simulink library "FMmodelBasic"  (R2022b)
settings: Solver=ode45  StartTime=0.0  StopTime=10.0  RelTol=1e-3  EnableMultiTasking=on
undefined symbols (not defined in the file or in its folder): aeroDB, envDB
libraries: utils x1
(part 1 of 2)
settings Model: Creator=Meyer-Brügel  LastModifiedBy=monas
settings SolverCC: AlgebraicLoopSolver=TrustRegion
settings DataIOCC: LimitDataPoints=on  SaveFormat=Array  ReturnWorkspaceOutputs=off
settings OptimizationCC: LifeSpan=inf
settings DebuggingCC: SolverPrmCheckMsg=warning  UnconnectedInputMsg=warning  UnconnectedOutputMsg=warning  UnconnectedLineMsg=warning  SFUnexpectedBacktrackingDiag=warning  SFNoUnconditionalDefaultTransitionDiag=warning  SFExecutionAtInitializationDiag=none  SFMachineParentedDataDiag=warning  ArithmeticOperatorsInVariantConditions=warning
settings HardwareCC: ProdBitPerPointer=32  ProdBitPerSizeT=32  ProdBitPerPtrDiffT=32  ProdLargestAtomicFloat=None  ProdIntDivRoundTo=Undefined  ProdEndianess=Unspecified  ProdWordSize=32  ProdHWDeviceType=32-bit Generic
settings ModelReferenceCC: EnableRefExpFcnMdlSchedulingChecks=on  PropagateSignalLabelsOutOfModel=off
settings SFSimCC: SimUseLocalCustomCode=off  CustomCodeUndefinedFunction=UseInterfaceOnly
settings RTWCC: RTWUseLocalCustomCode=off  DLArmComputeVersion=19.05
settings CodeAppCC: StateflowObjectComments=on
settings GRTTargetCC: TargetLangStandard=C89/C90 (ANSI)
settings ConfigComp: CovMetricSettings=dw  CovSaveCumulativeToWorkspaceVar=on  CovSaveSingleToWorkspaceVar=on  CovExternalEMLEnable=off  CovSFcnEnable=off

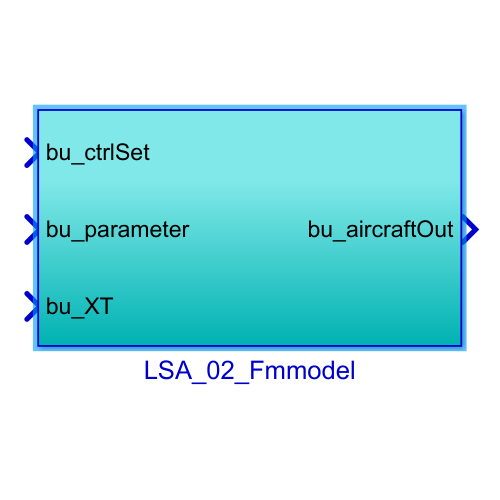
[thumbnail: Simulink's stored preview of the top-level diagram]
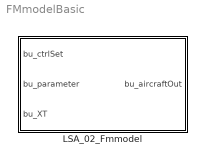
== system FMmodelBasic ==
  LSA_02_Fmmodel : Subsystem

== system FMmodelBasic/LSA_02_Fmmodel ==
  bu_ctrlSet : Inport  OutDataTypeStr=Bus: bu_ctrlSet
  bu_parameter : Inport  Port=2  OutDataTypeStr=Bus: bu_parameter
  bu_XT : Inport  Port=3  OutDataTypeStr=Bus: bu_XT
  Bus Creator : BusCreator  Inputs=3
  aircraft : Subsystem
  integrationProcces : Subsystem
  bu_aircraftOut : Outport  OutDataTypeStr=Bus: bu_aircraftOut
  wires:
  aircraft/1(bu_XaircraftDot) -> integrationProcces/2(bu_XaircraftDot), Bus Creator/2  "bu_XaircraftDot"
  aircraft/2(bu_aircraft) -> Bus Creator/3  "bu_aircraft"
  bu_ctrlSet/1 -> aircraft/2(bu_ctrlSet)
  integrationProcces/1("bu_Xaircraft ") -> aircraft/1("bu_Xaircraft "), Bus Creator/1  "bu_Xaircraft"
  Bus Creator/1 -> bu_aircraftOut/1  "bu_aircraftOut"
  bu_parameter/1 -> aircraft/3(bu_parameter)
  bu_XT/1 -> integrationProcces/1(bu_XT)

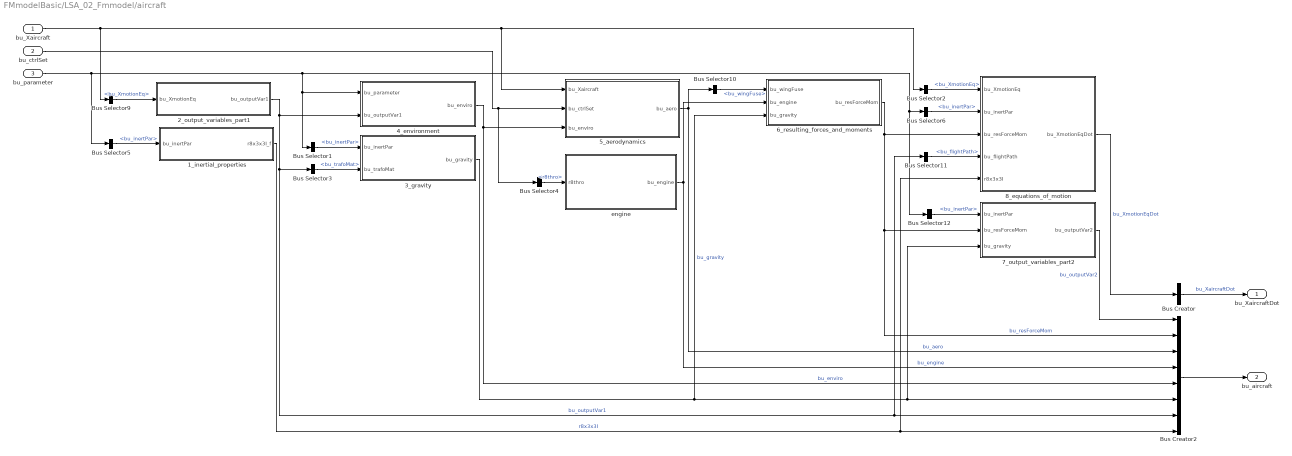
== system FMmodelBasic/LSA_02_Fmmodel/aircraft ==
  "bu_Xaircraft " : Inport
  bu_ctrlSet : Inport  Port=2
  bu_parameter : Inport  Port=3
  1_inertial_properties : Subsystem
  2_output_variables_part1 : Subsystem
  3_gravity : Subsystem
  4_environment : Subsystem
  5_aerodynamics : Subsystem
  6_resulting_forces_and_moments : Subsystem
  7_output_variables_part2 : Subsystem
  8_equations_of_motion : Subsystem
  Bus Creator : BusCreator  Inputs=1
  Bus Creator2 : BusCreator  Inputs=8
  Bus Selector{1,5..6,12} (4 alike) : BusSelector  OutputSignals=bu_inertPar
  Bus Selector10 : BusSelector  OutputSignals=bu_wingFuse
  Bus Selector11 : BusSelector  OutputSignals=bu_flightPath
  Bus Selector2 : BusSelector  OutputSignals=bu_XmotionEq
  Bus Selector3 : BusSelector  OutputSignals=bu_trafoMat
  Bus Selector4 : BusSelector  OutputSignals=r8thro
  Bus Selector9 : BusSelector  OutputSignals=bu_XmotionEq
  engine : Subsystem
  bu_XaircraftDot : Outport
  bu_aircraft : Outport  Port=2
  wires:
  Bus Creator/1 -> bu_XaircraftDot/1  "bu_XaircraftDot"
  Bus Creator2/1 -> bu_aircraft/1
  8_equations_of_motion/1(bu_XmotionEqDot) -> Bus Creator/1  "bu_XmotionEqDot"
  7_output_variables_part2/1(bu_outputVar2) -> Bus Creator2/1  "bu_outputVar2"
  6_resulting_forces_and_moments/1(bu_resForceMom) -> 8_equations_of_motion/3(bu_resForceMom), Bus Creator2/2, 7_output_variables_part2/2(bu_resForceMom)  "bu_resForceMom"
  5_aerodynamics/1(bu_aero) -> Bus Creator2/3, Bus Selector10/1  "bu_aero"
  Bus Selector2/1 -> 8_equations_of_motion/1(bu_XmotionEq)  "<bu_XmotionEq>"
  Bus Selector6/1 -> 8_equations_of_motion/2(bu_inertPar)  "<bu_inertPar>"
  Bus Selector10/1 -> 6_resulting_forces_and_moments/1(bu_wingFuse)  "<bu_wingFuse>"
  bu_ctrlSet/1 -> Bus Selector4/1, 5_aerodynamics/2(bu_ctrlSet)
  Bus Selector1/1 -> 3_gravity/1(bu_inertPar)  "<bu_inertPar>"
  Bus Selector3/1 -> 3_gravity/2(bu_trafoMat)  "<bu_trafoMat>"
  bu_parameter/1 -> Bus Selector12/1, Bus Selector6/1, Bus Selector1/1, 4_environment/1(bu_parameter), Bus Selector5/1
  Bus Selector5/1 -> 1_inertial_properties/1(bu_inertPar)  "<bu_inertPar>"
  "bu_Xaircraft "/1 -> Bus Selector9/1, 5_aerodynamics/1(bu_Xaircraft), Bus Selector2/1
  Bus Selector9/1 -> 2_output_variables_part1/1(bu_XmotionEq)  "<bu_XmotionEq>"
  Bus Selector11/1 -> 8_equations_of_motion/4(bu_flightPath)  "<bu_flightPath>"
  Bus Selector12/1 -> 7_output_variables_part2/1(bu_inertPar)  "<bu_inertPar>"
  2_output_variables_part1/1(bu_outputVar1) -> 4_environment/2(bu_outputVar1), Bus Selector3/1, Bus Selector11/1, Bus Creator2/7  "bu_outputVar1"
  3_gravity/1(bu_gravity) -> 6_resulting_forces_and_moments/3(bu_gravity), 7_output_variables_part2/3(bu_gravity), Bus Creator2/6  "bu_gravity"
  4_environment/1(bu_enviro) -> Bus Creator2/5, 5_aerodynamics/3(bu_enviro)  "bu_enviro"
  1_inertial_properties/1(r8x3x3I_f) -> 8_equations_of_motion/5(r8x3x3I), Bus Creator2/8  "r8x3x3I"
  Bus Selector4/1 -> engine/1(r8thro)  "<r8thro>"
  engine/1(bu_engine) -> Bus Creator2/4, 6_resulting_forces_and_moments/2(bu_engine)  "bu_engine"

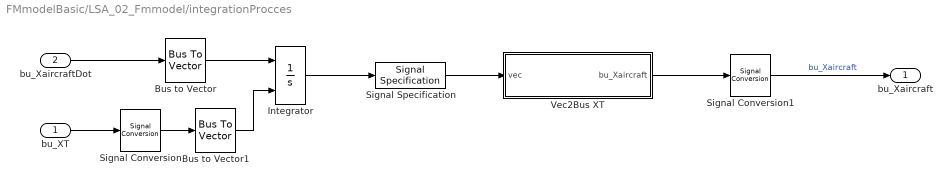
== system FMmodelBasic/LSA_02_Fmmodel/integrationProcces ==
  bu_XT : Inport
  bu_XaircraftDot : Inport  Port=2
  Bus to Vector : BusToVector
  Bus to Vector1 : BusToVector
  Integrator : Integrator  InitialConditionSource=external
  Signal Conversion : SignalConversion  ConversionOutput=Virtual bus  OverrideOpt=off
  Signal Conversion1 : SignalConversion  ConversionOutput=Virtual bus  OverrideOpt=off
  Signal Specification : SignalSpecification  Dimensions=[12,1]
  Vec2Bus XT : MATLAB Function  TreatAsAtomicUnit=on
  "bu_Xaircraft " : Outport
  wires:
  Bus to Vector/1 -> Integrator/1
  Integrator/1 -> Signal Specification/1
  bu_XaircraftDot/1 -> Bus to Vector/1
  bu_XT/1 -> Signal Conversion/1
  Signal Specification/1 -> Vec2Bus XT/1(vec)
  Bus to Vector1/1 -> Integrator/2
  Signal Conversion/1 -> Bus to Vector1/1
  Vec2Bus XT/1(bu_Xaircraft) -> Signal Conversion1/1
  Signal Conversion1/1 -> "bu_Xaircraft "/1  "bu_Xaircraft"

== system FMmodelBasic/LSA_02_Fmmodel/aircraft/1_inertial_properties ==
  bu_inertPar : Inport
  Bus Selector : BusSelector  OutputSignals=r8IOEWxx_f,r8IOEWyy_f,r8IOEWzz_f,r8IOEWxy_f,r8IOEWxz_f,r8IOEWyz_f
  MATLAB Function : MATLAB Function  TreatAsAtomicUnit=on
  r8x3x3I_f : Outport
  wires:
  bu_inertPar/1 -> Bus Selector/1
  Bus Selector/4 -> MATLAB Function/4(r8Ixy_f)  "<r8IOEWxy_f>"
  Bus Selector/6 -> MATLAB Function/6(r8Iyz_f)  "<r8IOEWyz_f>"
  Bus Selector/5 -> MATLAB Function/5(r8Ixz_f)  "<r8IOEWxz_f>"
  Bus Selector/3 -> MATLAB Function/3(r8Izz_f)  "<r8IOEWzz_f>"
  Bus Selector/2 -> MATLAB Function/2(r8Iyy_f)  "<r8IOEWyy_f>"
  Bus Selector/1 -> MATLAB Function/1(r8Ixx_f)  "<r8IOEWxx_f>"
  MATLAB Function/1(r8x3x3I_f) -> r8x3x3I_f/1  "r8x3x3I"

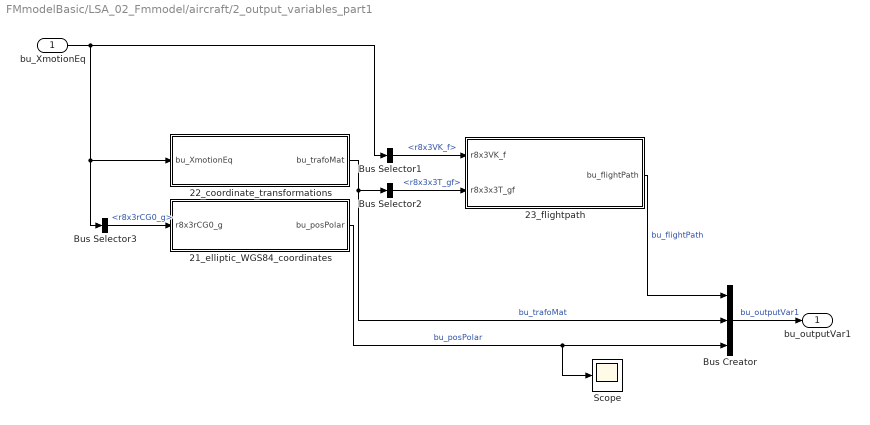
== system FMmodelBasic/LSA_02_Fmmodel/aircraft/2_output_variables_part1 ==
  bu_XmotionEq : Inport
  21_elliptic_WGS84_coordinates : Subsystem
  22_coordinate_transformations : Subsystem
  23_flightpath : Subsystem
  Bus Creator : BusCreator  Inputs=3
  Bus Selector1 : BusSelector  OutputSignals=r8x3VK_f
  Bus Selector2 : BusSelector  OutputSignals=r8x3x3T_gf
  Bus Selector3 : BusSelector  OutputSignals=r8x3rCG0_g
  Scope : Scope
  bu_outputVar1 : Outport
  wires:
  Bus Creator/1 -> bu_outputVar1/1  "bu_outputVar1"
  23_flightpath/1(bu_flightPath) -> Bus Creator/1  "bu_flightPath"
  22_coordinate_transformations/1(bu_trafoMat) -> Bus Creator/2, Bus Selector2/1  "bu_trafoMat"
  bu_XmotionEq/1 -> Bus Selector3/1, 22_coordinate_transformations/1(bu_XmotionEq), Bus Selector1/1
  Bus Selector1/1 -> 23_flightpath/1(r8x3VK_f)  "<r8x3VK_f>"
  Bus Selector2/1 -> 23_flightpath/2(r8x3x3T_gf)  "<r8x3x3T_gf>"
  21_elliptic_WGS84_coordinates/1(bu_posPolar) -> Scope/1, Bus Creator/3  "bu_posPolar"
  Bus Selector3/1 -> 21_elliptic_WGS84_coordinates/1(r8x3rCG0_g)  "<r8x3rCG0_g>"

== system FMmodelBasic/LSA_02_Fmmodel/aircraft/3_gravity ==
  bu_inertPar : Inport
  bu_trafoMat : Inport  Port=2
  31_gravity_g : Subsystem
  32_gravity_f : Subsystem
  Bus Creator1 : BusCreator  Inputs=2
  Bus Selector2 : BusSelector  OutputSignals=r8x3x3T_fg
  Bus Selector3 : BusSelector  OutputSignals=r8mOEW
  bu_gravity : Outport
  wires:
  Bus Creator1/1 -> bu_gravity/1  "bu_gravity"
  Bus Selector3/1 -> 31_gravity_g/1(r8mOEW)  "<r8mOEW>"
  bu_inertPar/1 -> Bus Selector3/1
  Bus Selector2/1 -> 32_gravity_f/1(r8x3x3T_fg)  "<r8x3x3T_fg>"
  bu_trafoMat/1 -> Bus Selector2/1
  32_gravity_f/1(r8x3G_f) -> Bus Creator1/1  "r8x3G_f"
  31_gravity_g/1(r8x3G_g) -> 32_gravity_f/2(r8x3G_g), Bus Creator1/2  "r8x3G_g"

== system FMmodelBasic/LSA_02_Fmmodel/aircraft/4_environment ==
  bu_parameter : Inport
  bu_outputVar1 : Inport  Port=2
  41_atmosphere : Subsystem
  Bus Creator : BusCreator  Inputs=1
  bu_enviro : Outport
  wires:
  Bus Creator/1 -> bu_enviro/1  "bu_enviro"
  41_atmosphere/1(bu_atmos) -> Bus Creator/1  "bu_atmos"
  bu_outputVar1/1 -> 41_atmosphere/2(bu_outputVar1)
  bu_parameter/1 -> 41_atmosphere/1(bu_parameter)

== system FMmodelBasic/LSA_02_Fmmodel/aircraft/5_aerodynamics ==
  bu_Xaircraft : Inport
  bu_ctrlSet : Inport  Port=2
  bu_enviro : Inport  Port=3
  51_effective_flow_at_ARP : Subsystem
  52_wing_and_fuselage : Subsystem
  Bus Creator : BusCreator  Inputs=2
  Bus Selector1 : BusSelector  OutputSignals=bu_XmotionEq
  Bus Selector2 : BusSelector  OutputSignals=bu_XmotionEq
  bu_aero : Outport
  wires:
  52_wing_and_fuselage/1(bu_wingFuse) -> Bus Creator/1  "bu_wingFuse"
  Bus Creator/1 -> bu_aero/1  "bu_aero"
  bu_Xaircraft/1 -> Bus Selector1/1, Bus Selector2/1
  bu_ctrlSet/1 -> 52_wing_and_fuselage/2(bu_ctrlSet)  "bu_ctrlSet"
  Bus Selector1/1 -> 52_wing_and_fuselage/1(bu_XmotionEq)  "<bu_XmotionEq>"
  Bus Selector2/1 -> 51_effective_flow_at_ARP/1(bu_XmotionEq)  "<bu_XmotionEq>"
  51_effective_flow_at_ARP/1(bu_effFlowARP) -> Bus Creator/2, 52_wing_and_fuselage/3(bu_effFlowARP)  "bu_effFlowARP"
  bu_enviro/1 -> 51_effective_flow_at_ARP/2(bu_enviro)

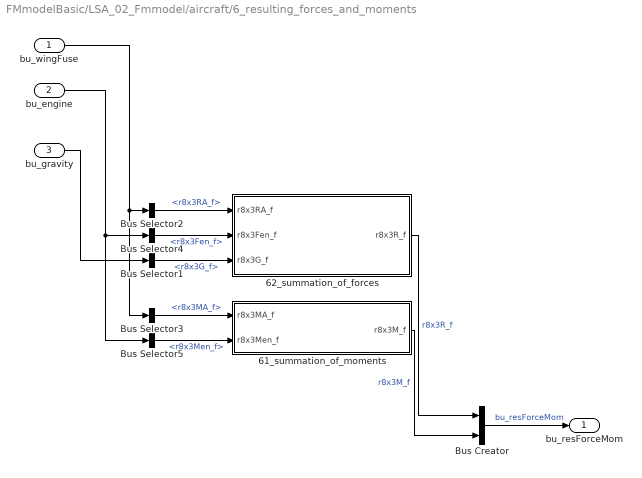
== system FMmodelBasic/LSA_02_Fmmodel/aircraft/6_resulting_forces_and_moments ==
  bu_wingFuse : Inport
  bu_engine : Inport  Port=2
  bu_gravity : Inport  Port=3
  61_summation_of_moments : Subsystem
  62_summation_of_forces : Subsystem
  Bus Creator : BusCreator  Inputs=2
  Bus Selector1 : BusSelector  OutputSignals=r8x3G_f
  Bus Selector2 : BusSelector  OutputSignals=bu_aeroForce.r8x3RA_f
  Bus Selector3 : BusSelector  OutputSignals=bu_aeroMoment.r8x3MA_f
  Bus Selector4 : BusSelector  OutputSignals=r8x3Fen_f
  Bus Selector5 : BusSelector  OutputSignals=r8x3Men_f
  bu_resForceMom : Outport
  wires:
  62_summation_of_forces/1(r8x3R_f) -> Bus Creator/1  "r8x3R_f"
  61_summation_of_moments/1("r8x3M_f ") -> Bus Creator/2  "r8x3M_f"
  Bus Creator/1 -> bu_resForceMom/1  "bu_resForceMom"
  Bus Selector2/1 -> 62_summation_of_forces/1(r8x3RA_f)  "<r8x3RA_f>"
  Bus Selector1/1 -> 62_summation_of_forces/3(r8x3G_f)  "<r8x3G_f>"
  Bus Selector3/1 -> 61_summation_of_moments/1(r8x3MA_f)  "<r8x3MA_f>"
  bu_wingFuse/1 -> Bus Selector3/1, Bus Selector2/1
  bu_gravity/1 -> Bus Selector1/1
  Bus Selector4/1 -> 62_summation_of_forces/2(r8x3Fen_f)  "<r8x3Fen_f>"
  bu_engine/1 -> Bus Selector4/1, Bus Selector5/1
  Bus Selector5/1 -> 61_summation_of_moments/2(r8x3Men_f)  "<r8x3Men_f>"

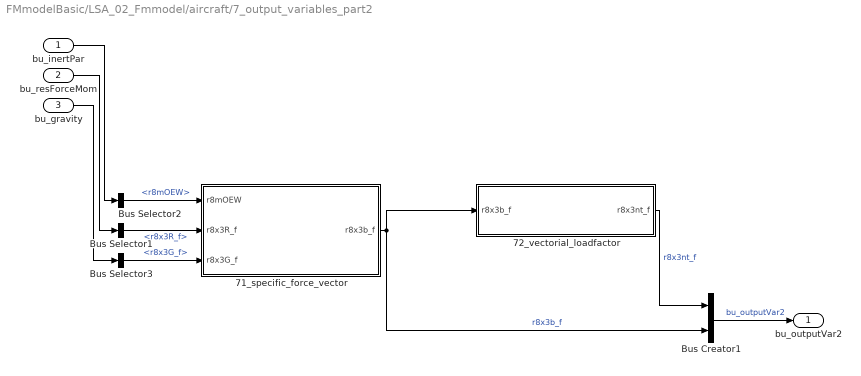
== system FMmodelBasic/LSA_02_Fmmodel/aircraft/7_output_variables_part2 ==
  bu_inertPar : Inport
  bu_resForceMom : Inport  Port=2
  bu_gravity : Inport  Port=3
  71_specific_force_vector : Subsystem
  72_vectorial_loadfactor : Subsystem
  Bus Creator1 : BusCreator  Inputs=2
  Bus Selector1 : BusSelector  OutputSignals=r8x3R_f
  Bus Selector2 : BusSelector  OutputSignals=r8mOEW
  Bus Selector3 : BusSelector  OutputSignals=r8x3G_f
  bu_outputVar2 : Outport
  wires:
  72_vectorial_loadfactor/1(r8x3nt_f) -> Bus Creator1/1  "r8x3nt_f"
  Bus Creator1/1 -> bu_outputVar2/1  "bu_outputVar2"
  Bus Selector2/1 -> 71_specific_force_vector/1(r8mOEW)  "<r8mOEW>"
  Bus Selector1/1 -> 71_specific_force_vector/2(r8x3R_f)  "<r8x3R_f>"
  Bus Selector3/1 -> 71_specific_force_vector/3(r8x3G_f)  "<r8x3G_f>"
  bu_inertPar/1 -> Bus Selector2/1
  bu_resForceMom/1 -> Bus Selector1/1
  bu_gravity/1 -> Bus Selector3/1
  71_specific_force_vector/1(r8x3b_f) -> 72_vectorial_loadfactor/1(r8x3b_f), Bus Creator1/2  "r8x3b_f"

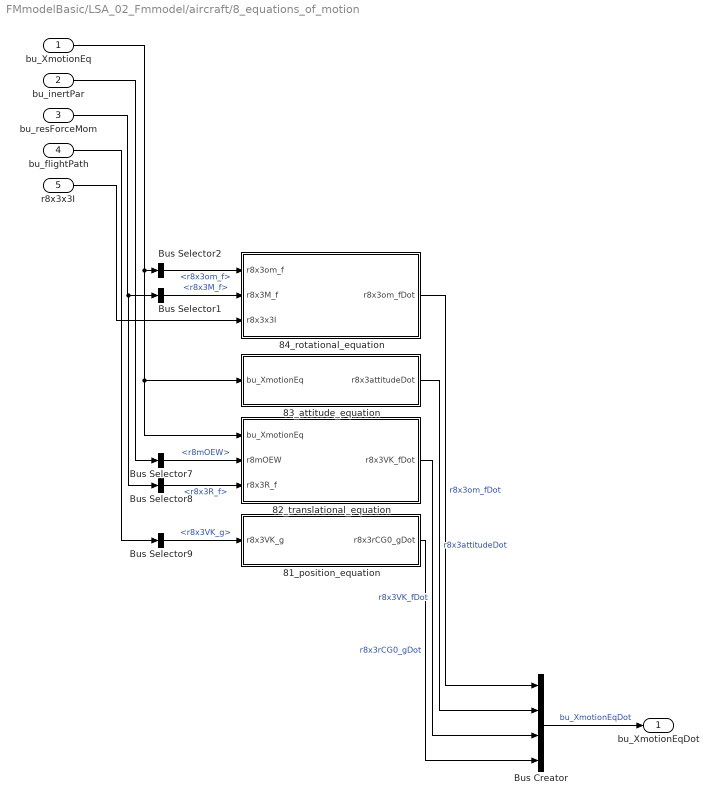
== system FMmodelBasic/LSA_02_Fmmodel/aircraft/8_equations_of_motion ==
  bu_XmotionEq : Inport
  bu_inertPar : Inport  Port=2
  bu_resForceMom : Inport  Port=3
  bu_flightPath : Inport  Port=4
  r8x3x3I : Inport  Port=5
  81_position_equation : Subsystem
  82_translational_equation : Subsystem
  83_attitude_equation : Subsystem
  84_rotational_equation : Subsystem
  Bus Creator : BusCreator  Inputs=4
  Bus Selector1 : BusSelector  OutputSignals=r8x3M_f
  Bus Selector2 : BusSelector  OutputSignals=r8x3om_f
  Bus Selector7 : BusSelector  OutputSignals=r8mOEW
  Bus Selector8 : BusSelector  OutputSignals=r8x3R_f
  Bus Selector9 : BusSelector  OutputSignals=r8x3VK_g
  bu_XmotionEqDot : Outport
  wires:
  Bus Creator/1 -> bu_XmotionEqDot/1  "bu_XmotionEqDot"
  Bus Selector2/1 -> 84_rotational_equation/1(r8x3om_f)  "<r8x3om_f>"
  Bus Selector1/1 -> 84_rotational_equation/2(r8x3M_f)  "<r8x3M_f>"
  bu_XmotionEq/1 -> 82_translational_equation/1(bu_XmotionEq), 83_attitude_equation/1(bu_XmotionEq), Bus Selector2/1
  bu_resForceMom/1 -> Bus Selector8/1, Bus Selector1/1
  r8x3x3I/1 -> 84_rotational_equation/3(r8x3x3I)
  Bus Selector7/1 -> 82_translational_equation/2(r8mOEW)  "<r8mOEW>"
  bu_inertPar/1 -> Bus Selector7/1
  Bus Selector8/1 -> 82_translational_equation/3(r8x3R_f)  "<r8x3R_f>"
  Bus Selector9/1 -> 81_position_equation/1(r8x3VK_g)  "<r8x3VK_g>"
  bu_flightPath/1 -> Bus Selector9/1
  84_rotational_equation/1(r8x3om_fDot) -> Bus Creator/1  "r8x3om_fDot"
  83_attitude_equation/1(r8x3attitudeDot) -> Bus Creator/2  "r8x3attitudeDot"
  82_translational_equation/1(r8x3VK_fDot) -> Bus Creator/3  "r8x3VK_fDot"
  81_position_equation/1(r8x3rCG0_gDot) -> Bus Creator/4  "r8x3rCG0_gDot"

== system FMmodelBasic/LSA_02_Fmmodel/aircraft/engine ==
  r8thro : Inport
  Bus Creator1 : BusCreator  Inputs=2
  Constant : Constant  Value=[1;0;0]  VectorParams1D=off
  Constant1 : Constant  Value=[0;0;0]  VectorParams1D=off
  Product : Product
  bu_engine : Outport
  wires:
  r8thro/1 -> Product/2
  Constant/1 -> Product/1
  Product/1 -> Bus Creator1/1  "r8x3Fen_f"
  Constant1/1 -> Bus Creator1/2  "r8x3Men_f"
  Bus Creator1/1 -> bu_engine/1  "bu_engine"

== system FMmodelBasic/LSA_02_Fmmodel/aircraft/2_output_variables_part1/21_elliptic_WGS84_coordinates ==
  r8x3rCG0_g : Inport
  Bus Creator : BusCreator  Inputs=3
  Demux : Demux  Outputs=3
  Divide : Product  Inputs=/*
  Fcn : Fcn  Expr=cos(u)*envDB.RE
  Gain : Gain  Gain=-1
  Gain1 : Gain  Gain=1/envDB.RE
  bu_posPolar : Outport
  wires:
  r8x3rCG0_g/1 -> Demux/1
  Bus Creator/1 -> bu_posPolar/1  "bu_posPolar"
  Demux/1 -> Gain1/1  "r8x_g"
  Demux/2 -> Divide/2  "r8y_g"
  Demux/3 -> Gain/1  "r8z_g"
  Gain/1 -> Bus Creator/3  "r8Hellip"
  Gain1/1 -> Bus Creator/1, Fcn/1  "r8lat"
  Divide/1 -> Bus Creator/2  "r8lon"
  Fcn/1 -> Divide/1

== system FMmodelBasic/LSA_02_Fmmodel/aircraft/2_output_variables_part1/22_coordinate_transformations ==
  bu_XmotionEq : Inport
  221_geodetic_to_bodyfixed : Subsystem
  222_bodyfixed_to_geodetic : Subsystem
  Bus Creator : BusCreator  Inputs=2
  Bus Selector5 : BusSelector  OutputSignals=r8x3attitude
  bu_trafoMat : Outport
  wires:
  bu_XmotionEq/1 -> Bus Selector5/1
  Bus Creator/1 -> bu_trafoMat/1  "bu_trafoMat"
  Bus Selector5/1 -> 221_geodetic_to_bodyfixed/1(r8x3attitude)  "<r8x3attitude>"
  222_bodyfixed_to_geodetic/1(r8x3x3T_gf) -> Bus Creator/1  "r8x3x3T_gf"
  221_geodetic_to_bodyfixed/1(r8x3x3T_fg) -> 222_bodyfixed_to_geodetic/1(r8x3x3T_fg), Bus Creator/2  "r8x3x3T_fg"

== system FMmodelBasic/LSA_02_Fmmodel/aircraft/2_output_variables_part1/23_flightpath ==
  r8x3VK_f : Inport
  r8x3x3T_gf : Inport  Port=2
  Bus Creator : BusCreator  Inputs=4
  MATLAB Function : MATLAB Function  TreatAsAtomicUnit=on
  Product : Product  Multiplication=Matrix(*)
  bu_flightPath : Outport
  wires:
  Bus Creator/1 -> bu_flightPath/1  "bu_flightPath"
  r8x3x3T_gf/1 -> Product/1
  Product/1 -> Bus Creator/4, MATLAB Function/1(r8x3VK_g)  "r8x3VK_g"
  r8x3VK_f/1 -> Product/2
  MATLAB Function/1(r8VK) -> Bus Creator/1  "r8VK"
  MATLAB Function/2(r8ga) -> Bus Creator/2  "r8ga"
  MATLAB Function/3(r8Ch) -> Bus Creator/3  "r8Ch"

== system FMmodelBasic/LSA_02_Fmmodel/aircraft/3_gravity/31_gravity_g ==
  r8mOEW : Inport
  Product : Product  RndMeth=Zero
  Vector Concatenate : Concatenate  NumInputs=3  Mode=Multidimensional array
  r8XG_g : Constant  Value=0
  r8YG_g : Constant  Value=0
  r8g : Constant  Value=envDB.g
  r8x3G_g : Outport
  wires:
  r8g/1 -> Product/2
  Product/1 -> Vector Concatenate/3
  r8XG_g/1 -> Vector Concatenate/1
  r8YG_g/1 -> Vector Concatenate/2
  r8mOEW/1 -> Product/1
  Vector Concatenate/1 -> r8x3G_g/1  "r8x3G_g"

== system FMmodelBasic/LSA_02_Fmmodel/aircraft/3_gravity/32_gravity_f ==
  r8x3x3T_fg : Inport
  r8x3G_g : Inport  Port=2
  Product1 : Product  Multiplication=Matrix(*)  RndMeth=Zero
  r8x3G_f : Outport
  wires:
  r8x3G_g/1 -> Product1/2
  Product1/1 -> r8x3G_f/1  "r8x3G_f"
  r8x3x3T_fg/1 -> Product1/1

== system FMmodelBasic/LSA_02_Fmmodel/aircraft/4_environment/41_atmosphere ==
  bu_parameter : Inport
  bu_outputVar1 : Inport  Port=2
  411_ISA_conditions : Subsystem
  412_wind : Subsystem
  Bus Creator1 : BusCreator  Inputs=2
  Bus Selector2 : BusSelector  OutputSignals=bu_trafoMat
  Bus Selector3 : BusSelector  OutputSignals=bu_posPolar.r8Hellip
  bu_atmos : Outport
  wires:
  411_ISA_conditions/1(bu_ISA) -> Bus Creator1/2  "bu_ISA"
  412_wind/1(bu_wind) -> Bus Creator1/1  "bu_wind"
  bu_parameter/1 -> 412_wind/1(bu_parameter)
  Bus Selector2/1 -> 412_wind/2(bu_trafoMat)  "<bu_trafoMat>"
  Bus Selector3/1 -> 411_ISA_conditions/1(r8Hellip)  "<r8Hellip>"
  bu_outputVar1/1 -> Bus Selector3/1, Bus Selector2/1
  Bus Creator1/1 -> bu_atmos/1  "bu_atmos"

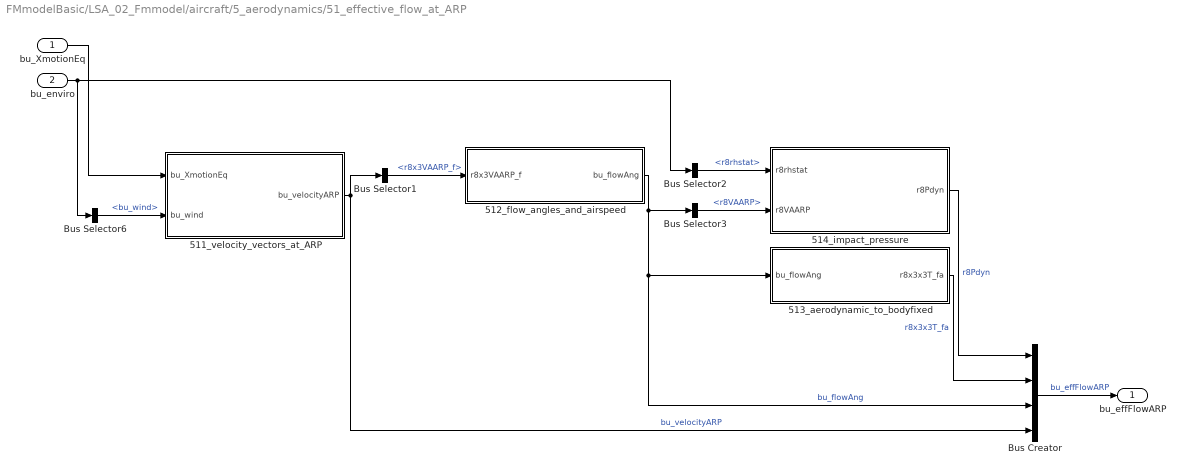
== system FMmodelBasic/LSA_02_Fmmodel/aircraft/5_aerodynamics/51_effective_flow_at_ARP ==
  bu_XmotionEq : Inport
  bu_enviro : Inport  Port=2
  511_velocity_vectors_at_ARP : Subsystem
  512_flow_angles_and_airspeed : Subsystem
  513_aerodynamic_to_bodyfixed : Subsystem
  514_impact_pressure : Subsystem
  Bus Creator : BusCreator  Inputs=4
  Bus Selector1 : BusSelector  OutputSignals=r8x3VAARP_f
  Bus Selector2 : BusSelector  OutputSignals=bu_atmos.bu_ISA.r8rhstat
  Bus Selector3 : BusSelector  OutputSignals=r8VAARP
  Bus Selector6 : BusSelector  OutputSignals=bu_atmos.bu_wind
  bu_effFlowARP : Outport
  wires:
  Bus Creator/1 -> bu_effFlowARP/1  "bu_effFlowARP"
  Bus Selector2/1 -> 514_impact_pressure/1(r8rhstat)  "<r8rhstat>"
  bu_XmotionEq/1 -> 511_velocity_vectors_at_ARP/1(bu_XmotionEq)
  bu_enviro/1 -> Bus Selector2/1, Bus Selector6/1
  Bus Selector1/1 -> 512_flow_angles_and_airspeed/1(r8x3VAARP_f)  "<r8x3VAARP_f>"
  511_velocity_vectors_at_ARP/1(bu_velocityARP) -> Bus Creator/4, Bus Selector1/1  "bu_velocityARP"
  Bus Selector3/1 -> 514_impact_pressure/2(r8VAARP)  "<r8VAARP>"
  512_flow_angles_and_airspeed/1(bu_flowAng) -> Bus Selector3/1, 513_aerodynamic_to_bodyfixed/1(bu_flowAng), Bus Creator/3  "bu_flowAng"
  513_aerodynamic_to_bodyfixed/1(r8x3x3T_fa) -> Bus Creator/2  "r8x3x3T_fa"
  514_impact_pressure/1(r8Pdyn) -> Bus Creator/1  "r8Pdyn"
  Bus Selector6/1 -> 511_velocity_vectors_at_ARP/2(bu_wind)  "<bu_wind>"

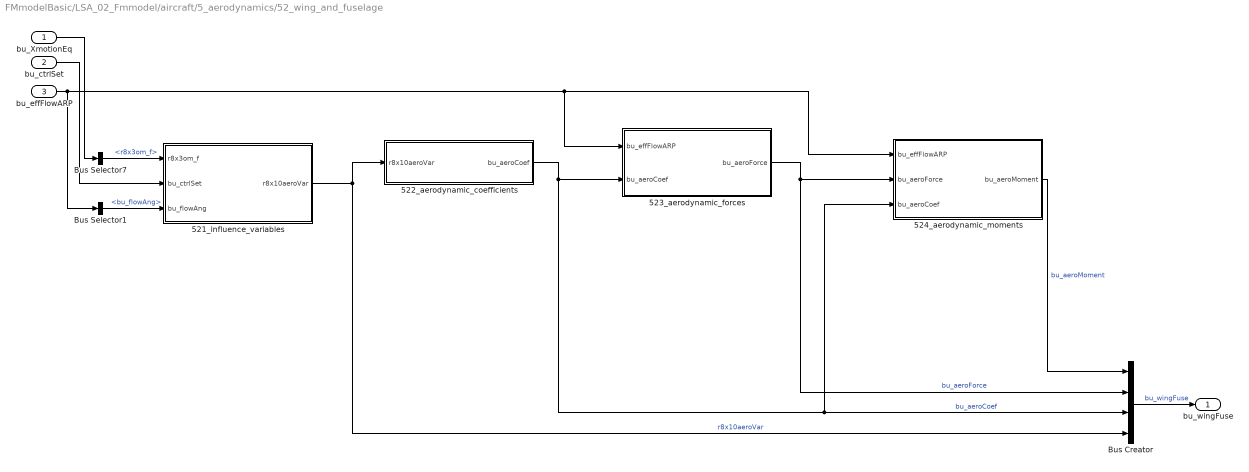
== system FMmodelBasic/LSA_02_Fmmodel/aircraft/5_aerodynamics/52_wing_and_fuselage ==
  bu_XmotionEq : Inport
  bu_ctrlSet : Inport  Port=2
  bu_effFlowARP : Inport  Port=3
  " 523_aerodynamic_forces" : Subsystem
  521_influence_variables : Subsystem
  522_aerodynamic_coefficients : Subsystem
  524_aerodynamic_moments : Subsystem
  Bus Creator : BusCreator  Inputs=4
  Bus Selector1 : BusSelector  OutputSignals=bu_flowAng
  Bus Selector7 : BusSelector  OutputSignals=r8x3om_f
  bu_wingFuse : Outport
  wires:
  Bus Creator/1 -> bu_wingFuse/1  "bu_wingFuse"
  Bus Selector7/1 -> 521_influence_variables/1(r8x3om_f)  "<r8x3om_f>"
  bu_XmotionEq/1 -> Bus Selector7/1
  bu_ctrlSet/1 -> 521_influence_variables/2(bu_ctrlSet)
  bu_effFlowARP/1 -> 524_aerodynamic_moments/1(bu_effFlowARP), " 523_aerodynamic_forces"/1(bu_effFlowARP), Bus Selector1/1
  524_aerodynamic_moments/1(bu_aeroMoment) -> Bus Creator/1  "bu_aeroMoment"
  " 523_aerodynamic_forces"/1(bu_aeroForce) -> 524_aerodynamic_moments/2(bu_aeroForce), Bus Creator/2  "bu_aeroForce"
  522_aerodynamic_coefficients/1(bu_aeroCoef) -> Bus Creator/3, 524_aerodynamic_moments/3(bu_aeroCoef), " 523_aerodynamic_forces"/2(bu_aeroCoef)  "bu_aeroCoef"
  521_influence_variables/1(r8x10aeroVar) -> 522_aerodynamic_coefficients/1(r8x10aeroVar), Bus Creator/4  "r8x10aeroVar"
  Bus Selector1/1 -> 521_influence_variables/3(bu_flowAng)  "<bu_flowAng>"

== system FMmodelBasic/LSA_02_Fmmodel/aircraft/6_resulting_forces_and_moments/61_summation_of_moments ==
  r8x3MA_f : Inport
  r8x3Men_f : Inport  Port=2
  Add : Sum
  "r8x3M_f " : Outport
  wires:
  Add/1 -> "r8x3M_f "/1
  r8x3MA_f/1 -> Add/1
  r8x3Men_f/1 -> Add/2

== system FMmodelBasic/LSA_02_Fmmodel/aircraft/6_resulting_forces_and_moments/62_summation_of_forces ==
  r8x3RA_f : Inport
  r8x3Fen_f : Inport  Port=2
  r8x3G_f : Inport  Port=3
  Add : Sum  Inputs=+++
  r8x3R_f : Outport
  wires:
  r8x3G_f/1 -> Add/3  "r8x3G_f"
  r8x3RA_f/1 -> Add/1  "r8x3RA_f"
  Add/1 -> r8x3R_f/1  "r8x3R_f"
  r8x3Fen_f/1 -> Add/2  "r8x3Fen_f"

== system FMmodelBasic/LSA_02_Fmmodel/aircraft/7_output_variables_part2/71_specific_force_vector ==
  r8mOEW : Inport
  r8x3R_f : Inport  Port=2
  r8x3G_f : Inport  Port=3
  Divide : Product  Inputs=/*
  Sum : Sum  Inputs=|+-
  r8x3b_f : Outport
  wires:
  r8x3R_f/1 -> Sum/1
  r8x3G_f/1 -> Sum/2
  Sum/1 -> Divide/2
  r8mOEW/1 -> Divide/1  "r8mOEW"
  Divide/1 -> r8x3b_f/1  "r8x3b_f"

== system FMmodelBasic/LSA_02_Fmmodel/aircraft/7_output_variables_part2/72_vectorial_loadfactor ==
  r8x3b_f : Inport
  Divide1 : Product  Inputs=*/
  r8g : Constant  Value=envDB.g
  r8x3nt_f : Outport
  wires:
  r8x3b_f/1 -> Divide1/1
  Divide1/1 -> r8x3nt_f/1  "r8x3nt_f"
  r8g/1 -> Divide1/2

== system FMmodelBasic/LSA_02_Fmmodel/aircraft/8_equations_of_motion/81_position_equation ==
  r8x3VK_g : Inport
  Gain : Gain
  r8x3rCG0_gDot : Outport
  wires:
  Gain/1 -> r8x3rCG0_gDot/1  "r8x3rCG0_gDot"
  r8x3VK_g/1 -> Gain/1  "r8x3VK_g"

== system FMmodelBasic/LSA_02_Fmmodel/aircraft/8_equations_of_motion/82_translational_equation ==
  bu_XmotionEq : Inport
  r8mOEW : Inport  Port=2
  r8x3R_f : Inport  Port=3
  Bus Selector5 : BusSelector  OutputSignals=r8x3om_f
  Bus Selector6 : BusSelector  OutputSignals=r8x3VK_f
  MATLAB Function : MATLAB Function  TreatAsAtomicUnit=on
  r8x3VK_fDot : Outport
  wires:
  MATLAB Function/1(r8x3VK_fDot) -> r8x3VK_fDot/1  "r8x3VK_fDot"
  r8mOEW/1 -> MATLAB Function/3(r8mOEW)  "r8mOEW"
  r8x3R_f/1 -> MATLAB Function/4(r8x3R_f)  "r8x3R_f"
  Bus Selector5/1 -> MATLAB Function/1(r8x3om_f)  "<r8x3om_f>"
  Bus Selector6/1 -> MATLAB Function/2(r8x3VK_f)  "<r8x3VK_f>"
  bu_XmotionEq/1 -> Bus Selector6/1, Bus Selector5/1

== system FMmodelBasic/LSA_02_Fmmodel/aircraft/8_equations_of_motion/83_attitude_equation ==
  bu_XmotionEq : Inport
  Bus Selector3 : BusSelector  OutputSignals=r8x3attitude,r8x3om_f
  MATLAB Function : MATLAB Function  TreatAsAtomicUnit=on
  r8x3attitudeDot : Outport
  wires:
  bu_XmotionEq/1 -> Bus Selector3/1
  Bus Selector3/1 -> MATLAB Function/1(r8x3attitude)  "<r8x3attitude>"
  MATLAB Function/1(r8x3attitudeDot) -> r8x3attitudeDot/1
  Bus Selector3/2 -> MATLAB Function/2(r8x3om_f)  "<r8x3om_f>"

== system FMmodelBasic/LSA_02_Fmmodel/aircraft/8_equations_of_motion/84_rotational_equation ==
  r8x3om_f : Inport
  r8x3M_f : Inport  Port=2
  r8x3x3I : Inport  Port=3
  MATLAB Function : MATLAB Function  TreatAsAtomicUnit=on
  r8x3om_fDot : Outport
  wires:
  r8x3om_f/1 -> MATLAB Function/1(r8x3om_f)  "r8x3om_f"
  r8x3x3I/1 -> MATLAB Function/2(r8x3x3I_f)
  MATLAB Function/1(r8x3om_fDot) -> r8x3om_fDot/1  "r8x3om_fDot"
  r8x3M_f/1 -> MATLAB Function/3(r8x3M_f)  "r8x3M_f"

== system FMmodelBasic/LSA_02_Fmmodel/aircraft/2_output_variables_part1/22_coordinate_transformations/221_geodetic_to_bodyfixed ==
  r8x3attitude : Inport
  Tfg : MATLAB Function  TreatAsAtomicUnit=on
  r8x3x3T_fg : Outport  OutDataTypeStr=double  PortDimensions=[3 3]
  wires:
  r8x3attitude/1 -> Tfg/1(r8x3attitude)
  Tfg/1(r8T_fg) -> r8x3x3T_fg/1  "r8x3x3T_fg"

== system FMmodelBasic/LSA_02_Fmmodel/aircraft/2_output_variables_part1/22_coordinate_transformations/222_bodyfixed_to_geodetic ==
  r8x3x3T_fg : Inport
  Math Function : Math  Operator=transpose  SignedPower=on
  r8x3x3T_gf : Outport
  wires:
  r8x3x3T_fg/1 -> Math Function/1
  Math Function/1 -> r8x3x3T_gf/1  "r8x3x3T_gf"

== system FMmodelBasic/LSA_02_Fmmodel/aircraft/4_environment/41_atmosphere/411_ISA_conditions ==
  r8Hellip : Inport
  4111_geopotential_height : Subsystem
  4112_static_temperature : Subsystem
  4113_static_pressure : Subsystem
  4114_static_density : Subsystem
  Bus Creator : BusCreator  Inputs=6
  bu_ISA : Outport
  wires:
  Bus Creator/1 -> bu_ISA/1  "bu_ISA"
  r8Hellip/1 -> 4111_geopotential_height/1(r8h)
  4111_geopotential_height/1(r8H) -> 4112_static_temperature/1(r8H), 4113_static_pressure/3(r8H), Bus Creator/6  "r8H"
  4112_static_temperature/3(ui4_ISAfraction) -> Bus Creator/5  "ui4_ISAwidth"
  4112_static_temperature/2(ui4_ISAsegment) -> 4113_static_pressure/2(ui4_ISAsegment), Bus Creator/4  "ui4_ISAsegment"
  4112_static_temperature/1(r8Tstat) -> 4114_static_density/2(r8Tstat), Bus Creator/3, 4113_static_pressure/1(r8Tstat)  "r8Tstat"
  4113_static_pressure/1(r8Pstat) -> 4114_static_density/1(r8Pstat), Bus Creator/2  "r8Pstat"
  4114_static_density/1(r8rhstat) -> Bus Creator/1  "r8rhstat"

== system FMmodelBasic/LSA_02_Fmmodel/aircraft/4_environment/41_atmosphere/412_wind ==
  bu_parameter : Inport
  bu_trafoMat : Inport  Port=2
  4121_windVelocity_g : Subsystem
  4122_windVelocity_f : Subsystem
  Bus Creator1 : BusCreator  Inputs=2
  Bus Selector1 : BusSelector  OutputSignals=bu_windPar
  Bus Selector14 : BusSelector  OutputSignals=r8x3x3T_fg
  bu_wind : Outport
  wires:
  bu_parameter/1 -> Bus Selector1/1
  Bus Selector14/1 -> 4122_windVelocity_f/1(r8x3x3T_fg)  "<r8x3x3T_fg>"
  bu_trafoMat/1 -> Bus Selector14/1
  4122_windVelocity_f/1(r8x3VW_f) -> Bus Creator1/1  "r8x3VW_f"
  4121_windVelocity_g/1(r8x3VW_g) -> Bus Creator1/2, 4122_windVelocity_f/2(r8x3VW_g)  "r8x3VW_g"
  Bus Creator1/1 -> bu_wind/1  "bu_wind"
  Bus Selector1/1 -> 4121_windVelocity_g/1(bu_windPar)  "<bu_windPar>"

== system FMmodelBasic/LSA_02_Fmmodel/aircraft/5_aerodynamics/51_effective_flow_at_ARP/511_velocity_vectors_at_ARP ==
  bu_XmotionEq : Inport
  bu_wind : Inport  Port=2
  5111_path_velocity_at_ARP : Subsystem
  5112_flow_velocity_at_ARP : Subsystem
  Bus Creator1 : BusCreator  Inputs=2
  Bus Selector3 : BusSelector  OutputSignals=r8x3VW_f
  bu_velocityARP : Outport
  wires:
  Bus Selector3/1 -> 5112_flow_velocity_at_ARP/1(r8x3VW_f)  "<r8x3VW_f>"
  bu_wind/1 -> Bus Selector3/1
  Bus Creator1/1 -> bu_velocityARP/1  "bu_velocityARP"
  5111_path_velocity_at_ARP/1(r8x3VKARP_f) -> 5112_flow_velocity_at_ARP/2(r8x3VKARP_f), Bus Creator1/2  "r8x3VKARP_f"
  5112_flow_velocity_at_ARP/1(r8x3VAARP_f) -> Bus Creator1/1  "r8x3VAARP_f"
  bu_XmotionEq/1 -> 5111_path_velocity_at_ARP/1(bu_XmotionEq)  "bu_XmotionEq"

== system FMmodelBasic/LSA_02_Fmmodel/aircraft/5_aerodynamics/51_effective_flow_at_ARP/512_flow_angles_and_airspeed ==
  r8x3VAARP_f : Inport
  Bus Creator : BusCreator  Inputs=3
  MATLAB Function : MATLAB Function  TreatAsAtomicUnit=on
  bu_flowAng : Outport
  wires:
  MATLAB Function/1(r8alARP) -> Bus Creator/1  "r8alARP"
  MATLAB Function/2(r8beARP) -> Bus Creator/2  "r8beARP"
  Bus Creator/1 -> bu_flowAng/1  "bu_flowAng"
  r8x3VAARP_f/1 -> MATLAB Function/1(r8x3VAARP_f)
  MATLAB Function/3(r8VAARP) -> Bus Creator/3  "r8VAARP"

== system FMmodelBasic/LSA_02_Fmmodel/aircraft/5_aerodynamics/51_effective_flow_at_ARP/513_aerodynamic_to_bodyfixed ==
  bu_flowAng : Inport
  Bus Selector4 : BusSelector  OutputSignals=r8alARP
  Bus Selector5 : BusSelector  OutputSignals=r8beARP
  Tfa : MATLAB Function  TreatAsAtomicUnit=on
  r8x3x3T_fa : Outport
  wires:
  Tfa/1(r8T_fa) -> r8x3x3T_fa/1  "r8x3x3T_fa"
  Bus Selector4/1 -> Tfa/1(r8alARP)  "<r8alARP>"
  Bus Selector5/1 -> Tfa/2(r8beARP)  "<r8beARP>"
  bu_flowAng/1 -> Bus Selector5/1, Bus Selector4/1

== system FMmodelBasic/LSA_02_Fmmodel/aircraft/5_aerodynamics/51_effective_flow_at_ARP/514_impact_pressure ==
  r8rhstat : Inport
  r8VAARP : Inport  Port=2
  Gain : Gain  Gain=0.5
  Math Function : Math  Operator=square  SignedPower=on
  Product : Product
  To Workspace : ToWorkspace  VariableName=rho_stat  SaveFormat=Timeseries  SampleTime=-1
  r8Pdyn : Outport
  wires:
  Product/1 -> r8Pdyn/1  "r8Pdyn"
  r8VAARP/1 -> Math Function/1
  r8rhstat/1 -> To Workspace/1, Gain/1
  Gain/1 -> Product/1
  Math Function/1 -> Product/2

== system FMmodelBasic/LSA_02_Fmmodel/aircraft/5_aerodynamics/52_wing_and_fuselage/ 523_aerodynamic_forces ==
  bu_effFlowARP : Inport
  bu_aeroCoef : Inport  Port=2
  5231_in_aerodynamic_coordinates : Subsystem
  5232_in_body_fixed_coordinates : Subsystem
  Bus Creator1 : BusCreator  Inputs=2
  Bus Selector1 : BusSelector  OutputSignals=r8x3forceCoef
  Bus Selector4 : BusSelector  OutputSignals=r8x3x3T_fa
  Bus Selector7 : BusSelector  OutputSignals=r8Pdyn
  bu_aeroForce : Outport
  wires:
  Bus Selector7/1 -> 5231_in_aerodynamic_coordinates/1(r8Pdyn)  "<r8Pdyn>"
  Bus Selector1/1 -> 5231_in_aerodynamic_coordinates/2(r8x3forceCoef)  "<r8x3forceCoef>"
  bu_aeroCoef/1 -> Bus Selector1/1
  bu_effFlowARP/1 -> Bus Selector7/1, Bus Selector4/1
  Bus Selector4/1 -> 5232_in_body_fixed_coordinates/1(r8x3x3T_fa)  "<r8x3x3T_fa>"
  Bus Creator1/1 -> bu_aeroForce/1  "bu_aeroForce"
  5232_in_body_fixed_coordinates/1(r8x3RA_f) -> Bus Creator1/1  "r8x3RA_f"
  5231_in_aerodynamic_coordinates/1(r8x3RA_a) -> Bus Creator1/2, 5232_in_body_fixed_coordinates/2(r8x3RA_a)  "r8x3RA_a"

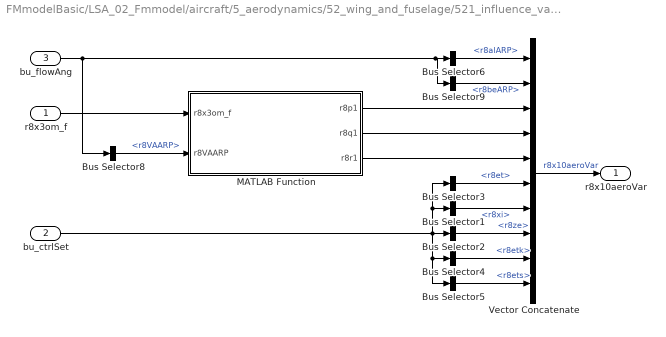
== system FMmodelBasic/LSA_02_Fmmodel/aircraft/5_aerodynamics/52_wing_and_fuselage/521_influence_variables ==
  r8x3om_f : Inport
  bu_ctrlSet : Inport  Port=2
  bu_flowAng : Inport  Port=3
  Bus Selector1 : BusSelector  OutputSignals=r8xi
  Bus Selector2 : BusSelector  OutputSignals=r8ze
  Bus Selector3 : BusSelector  OutputSignals=r8et
  Bus Selector4 : BusSelector  OutputSignals=r8etk
  Bus Selector5 : BusSelector  OutputSignals=r8ets
  Bus Selector6 : BusSelector  OutputSignals=r8alARP
  Bus Selector8 : BusSelector  OutputSignals=r8VAARP
  Bus Selector9 : BusSelector  OutputSignals=r8beARP
  MATLAB Function : MATLAB Function  TreatAsAtomicUnit=on
  Vector Concatenate : Concatenate  NumInputs=10  Mode=Multidimensional array
  r8x10aeroVar : Outport
  wires:
  Vector Concatenate/1 -> r8x10aeroVar/1  "r8x10aeroVar"
  MATLAB Function/1(r8p1) -> Vector Concatenate/3
  MATLAB Function/2(r8q1) -> Vector Concatenate/4
  MATLAB Function/3(r8r1) -> Vector Concatenate/5
  r8x3om_f/1 -> MATLAB Function/1(r8x3om_f)
  bu_flowAng/1 -> Bus Selector9/1, Bus Selector6/1, Bus Selector8/1
  Bus Selector3/1 -> Vector Concatenate/6  "<r8et>"
  Bus Selector1/1 -> Vector Concatenate/7  "<r8xi>"
  Bus Selector2/1 -> Vector Concatenate/8  "<r8ze>"
  Bus Selector4/1 -> Vector Concatenate/9  "<r8etk>"
  Bus Selector5/1 -> Vector Concatenate/10  "<r8ets>"
  Bus Selector6/1 -> Vector Concatenate/1  "<r8alARP>"
  Bus Selector8/1 -> MATLAB Function/2(r8VAARP)  "<r8VAARP>"
  Bus Selector9/1 -> Vector Concatenate/2  "<r8beARP>"
  bu_ctrlSet/1 -> Bus Selector3/1, Bus Selector1/1, Bus Selector5/1, Bus Selector4/1, Bus Selector2/1

== system FMmodelBasic/LSA_02_Fmmodel/aircraft/5_aerodynamics/52_wing_and_fuselage/522_aerodynamic_coefficients ==
  r8x10aeroVar : Inport
  Bus Creator1 : BusCreator  Inputs=2
  MATLAB Function : MATLAB Function  TreatAsAtomicUnit=on
  Math Function : Math  Operator=transpose  SignedPower=on
  To Workspace : ToWorkspace  VariableName=aero_coeff  SaveFormat=Timeseries  SampleTime=-1
  bu_aeroCoef : Outport
  wires:
  r8x10aeroVar/1 -> Math Function/1
  Bus Creator1/1 -> To Workspace/1, bu_aeroCoef/1  "bu_aeroCoef"
  Math Function/1 -> MATLAB Function/1(AeroVar)
  MATLAB Function/1(r8x3forceCoef) -> Bus Creator1/1  "r8x3forceCoef"
  MATLAB Function/2(r8x3momentCoef) -> Bus Creator1/2  "r8x3momentCoef"

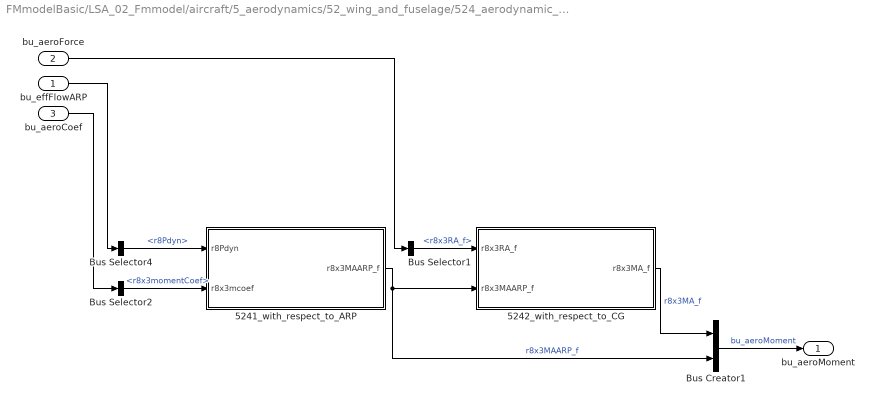
== system FMmodelBasic/LSA_02_Fmmodel/aircraft/5_aerodynamics/52_wing_and_fuselage/524_aerodynamic_moments ==
  bu_effFlowARP : Inport
  bu_aeroForce : Inport  Port=2
  bu_aeroCoef : Inport  Port=3
  5241_with_respect_to_ARP : Subsystem
  5242_with_respect_to_CG : Subsystem
  Bus Creator1 : BusCreator  Inputs=2
  Bus Selector1 : BusSelector  OutputSignals=r8x3RA_f
  Bus Selector2 : BusSelector  OutputSignals=r8x3momentCoef
  Bus Selector4 : BusSelector  OutputSignals=r8Pdyn
  bu_aeroMoment : Outport
  wires:
  5242_with_respect_to_CG/1(r8x3MA_f) -> Bus Creator1/1  "r8x3MA_f"
  Bus Creator1/1 -> bu_aeroMoment/1  "bu_aeroMoment"
  Bus Selector1/1 -> 5242_with_respect_to_CG/1(r8x3RA_f)  "<r8x3RA_f>"
  Bus Selector2/1 -> 5241_with_respect_to_ARP/2(r8x3mcoef)  "<r8x3momentCoef>"
  bu_aeroForce/1 -> Bus Selector1/1
  Bus Selector4/1 -> 5241_with_respect_to_ARP/1(r8Pdyn)  "<r8Pdyn>"
  bu_effFlowARP/1 -> Bus Selector4/1
  bu_aeroCoef/1 -> Bus Selector2/1
  5241_with_respect_to_ARP/1(r8x3MAARP_f) -> Bus Creator1/2, 5242_with_respect_to_CG/2(r8x3MAARP_f)  "r8x3MAARP_f"

== system FMmodelBasic/LSA_02_Fmmodel/aircraft/4_environment/41_atmosphere/411_ISA_conditions/4111_geopotential_height ==
  r8h : Inport
  1 : Constant
  Constant : Constant  Value=0
  Divide : Product  Inputs=*/
  Divide1 : Product  Inputs=*/
  Manual Switch : ManualSwitch  CurrentSetting=0
  Sum : Sum  Inputs=|++
  r8RE : Constant  Value=envDB.RE
  r8H : Outport
  wires:
  Manual Switch/1 -> r8H/1  "r8H"
  Divide/1 -> Sum/1
  1/1 -> Sum/2
  r8h/1 -> Divide/1, Divide1/1
  Sum/1 -> Divide1/2
  r8RE/1 -> Divide/2
  Constant/1 -> Manual Switch/1
  Divide1/1 -> Manual Switch/2  "r8H"

== system FMmodelBasic/LSA_02_Fmmodel/aircraft/4_environment/41_atmosphere/411_ISA_conditions/4112_static_temperature ==
  r8H : Inport
  prelookupIntr : Interpolation_n-D  NumberOfTableDimensions=1  Table=envDB.T
      settings: InputPortMap=u0,u1
  prelookup_T : PreLookup  BreakpointsData=envDB.H  ExtrapMethod=Linear
  r8Tstat : Outport
  ui4_ISAsegment : Outport  Port=2
  ui4_ISAfraction : Outport  Port=3
  wires:
  prelookupIntr/1 -> r8Tstat/1  "r8Tstat"
  prelookup_T/2 -> prelookupIntr/2, ui4_ISAfraction/1  "ui4_ISAfraction"
  prelookup_T/1 -> prelookupIntr/1, ui4_ISAsegment/1  "ui4_ISAsegment"
  r8H/1 -> prelookup_T/1

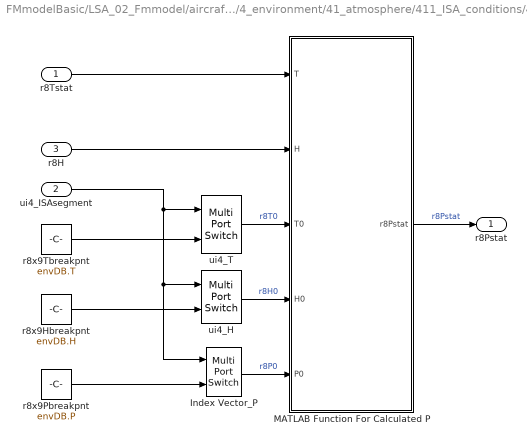
== system FMmodelBasic/LSA_02_Fmmodel/aircraft/4_environment/41_atmosphere/411_ISA_conditions/4113_static_pressure ==
  r8Tstat : Inport
  ui4_ISAsegment : Inport  Port=2
  r8H : Inport  Port=3
  Index Vector_P : MultiPortSwitch  DataPortOrder=Zero-based contiguous  Inputs=1  zeroidx=on  SaturateOnIntegerOverflow=off  InputSameDT=off
  MATLAB Function For Calculated P : MATLAB Function  TreatAsAtomicUnit=on
  r8x9Hbreakpnt : Constant  Value=envDB.H
  r8x9Pbreakpnt : Constant  Value=envDB.P
  r8x9Tbreakpnt : Constant  Value=envDB.T
  ui4_H : MultiPortSwitch  DataPortOrder=Zero-based contiguous  Inputs=1  zeroidx=on  SaturateOnIntegerOverflow=off  InputSameDT=off
  ui4_T : MultiPortSwitch  DataPortOrder=Zero-based contiguous  Inputs=1  zeroidx=on  SaturateOnIntegerOverflow=off  InputSameDT=off
  r8Pstat : Outport
  wires:
  r8H/1 -> MATLAB Function For Calculated P/2(H)
  r8x9Pbreakpnt/1 -> Index Vector_P/2
  Index Vector_P/1 -> MATLAB Function For Calculated P/5(P0)  "r8P0"
  r8x9Tbreakpnt/1 -> ui4_T/2
  ui4_T/1 -> MATLAB Function For Calculated P/3(T0)  "r8T0"
  MATLAB Function For Calculated P/1(r8Pstat) -> r8Pstat/1  "r8Pstat"
  ui4_H/1 -> MATLAB Function For Calculated P/4(H0)  "r8H0"
  r8x9Hbreakpnt/1 -> ui4_H/2
  ui4_ISAsegment/1 -> ui4_T/1, Index Vector_P/1, ui4_H/1
  r8Tstat/1 -> MATLAB Function For Calculated P/1(T)

== system FMmodelBasic/LSA_02_Fmmodel/aircraft/4_environment/41_atmosphere/411_ISA_conditions/4114_static_density ==
  r8Pstat : Inport
  r8Tstat : Inport  Port=2
  Divide : Product  Inputs=*/
  Product : Product  RndMeth=Zero
  r8R : Constant  Value=envDB.R
  r8rhstat : Outport
  wires:
  r8R/1 -> Product/2
  Product/1 -> Divide/2
  r8Pstat/1 -> Divide/1
  r8Tstat/1 -> Product/1  "r8Tstat"
  Divide/1 -> r8rhstat/1  "r8rhstat"

== system FMmodelBasic/LSA_02_Fmmodel/aircraft/4_environment/41_atmosphere/412_wind/4121_windVelocity_g ==
  bu_windPar : Inport
  Bus Selector1 : BusSelector  OutputSignals=r8ChW
  Bus Selector14 : BusSelector  OutputSignals=r8gaW
  Bus Selector2 : BusSelector  OutputSignals=r8VW
  MATLAB Function : MATLAB Function  TreatAsAtomicUnit=on
  r8x3VW_g : Outport
  wires:
  MATLAB Function/1(r8x3VW_g) -> r8x3VW_g/1  "r8x3VW_g"
  bu_windPar/1 -> Bus Selector14/1, Bus Selector1/1, Bus Selector2/1
  Bus Selector14/1 -> MATLAB Function/1(r8gaW)  "<r8gaW>"
  Bus Selector1/1 -> MATLAB Function/2(r8ChW)  "<r8ChW>"
  Bus Selector2/1 -> MATLAB Function/3(r8VW)  "<r8VW>"

== system FMmodelBasic/LSA_02_Fmmodel/aircraft/4_environment/41_atmosphere/412_wind/4122_windVelocity_f ==
  r8x3x3T_fg : Inport
  r8x3VW_g : Inport  Port=2
  Product1 : Product  Multiplication=Matrix(*)  RndMeth=Zero
  r8x3VW_f : Outport
  wires:
  r8x3VW_g/1 -> Product1/2
  r8x3x3T_fg/1 -> Product1/1
  Product1/1 -> r8x3VW_f/1  "r8x3VW_f"

== system FMmodelBasic/LSA_02_Fmmodel/aircraft/5_aerodynamics/51_effective_flow_at_ARP/511_velocity_vectors_at_ARP/5111_path_velocity_at_ARP ==
  bu_XmotionEq : Inport
  Bus Selector1 : BusSelector  OutputSignals=r8x3VK_f
  Bus Selector2 : BusSelector  OutputSignals=r8x3om_f
  Constant : Constant  Value=[aeroDB.xARP_f;aeroDB.yARP_f;aeroDB.zARP_f]  VectorParams1D=off
  Sum : Sum  Inputs=|++
  "cross " : utils/cross 
  r8x3VKARP_f : Outport
  wires:
  "cross "/1 -> Sum/1
  Sum/1 -> r8x3VKARP_f/1  "r8x3VKARP_f"
  bu_XmotionEq/1 -> Bus Selector1/1, Bus Selector2/1
  Bus Selector2/1 -> "cross "/1  "<r8x3om_f>"
  Bus Selector1/1 -> Sum/2  "<r8x3VK_f>"
  Constant/1 -> "cross "/2

== system FMmodelBasic/LSA_02_Fmmodel/aircraft/5_aerodynamics/51_effective_flow_at_ARP/511_velocity_vectors_at_ARP/5112_flow_velocity_at_ARP ==
  r8x3VW_f : Inport
  r8x3VKARP_f : Inport  Port=2
  Add1 : Sum
  r8x3VAARP_f : Outport
  wires:
  Add1/1 -> r8x3VAARP_f/1  "r8x3VAARP_f"
  r8x3VKARP_f/1 -> Add1/2
  r8x3VW_f/1 -> Add1/1

== system FMmodelBasic/LSA_02_Fmmodel/aircraft/5_aerodynamics/52_wing_and_fuselage/ 523_aerodynamic_forces/5231_in_aerodynamic_coordinates ==
  r8Pdyn : Inport
  r8x3forceCoef : Inport  Port=2
  MATLAB Function : MATLAB Function  TreatAsAtomicUnit=on
  r8x3RA_a : Outport
  wires:
  MATLAB Function/1(r8x3RA_a) -> r8x3RA_a/1  "r8x3RA_a"
  r8x3forceCoef/1 -> MATLAB Function/2(r8x3forceCoef)
  r8Pdyn/1 -> MATLAB Function/1(r8Pdyn)

== system FMmodelBasic/LSA_02_Fmmodel/aircraft/5_aerodynamics/52_wing_and_fuselage/ 523_aerodynamic_forces/5232_in_body_fixed_coordinates ==
  r8x3x3T_fa : Inport
  r8x3RA_a : Inport  Port=2
  Product2 : Product  Multiplication=Matrix(*)  RndMeth=Zero
  r8x3RA_f : Outport
  wires:
  r8x3RA_a/1 -> Product2/2
  Product2/1 -> r8x3RA_f/1  "r8x3RA_f"
  r8x3x3T_fa/1 -> Product2/1

== system FMmodelBasic/LSA_02_Fmmodel/aircraft/5_aerodynamics/52_wing_and_fuselage/524_aerodynamic_moments/5241_with_respect_to_ARP ==
  r8Pdyn : Inport
  r8x3mcoef : Inport  Port=2
  MATLAB Function : MATLAB Function  TreatAsAtomicUnit=on
  r8x3MAARP_f : Outport
  wires:
  MATLAB Function/1(r8x3MAARP_f) -> r8x3MAARP_f/1  "r8x3MAARP_f"
  r8Pdyn/1 -> MATLAB Function/1(r8Pdyn)
  r8x3mcoef/1 -> MATLAB Function/2(r8x3mcoef)

== system FMmodelBasic/LSA_02_Fmmodel/aircraft/5_aerodynamics/52_wing_and_fuselage/524_aerodynamic_moments/5242_with_respect_to_CG ==
  r8x3RA_f : Inport
  r8x3MAARP_f : Inport  Port=2
  MATLAB Function : MATLAB Function  TreatAsAtomicUnit=on
  Sum : Sum  Inputs=|++  AccumDataTypeStr=double  OutDataTypeStr=double
  r8x3MA_f : Outport
  wires:
  Sum/1 -> r8x3MA_f/1  "r8x3MA_f"
  MATLAB Function/1(r8x3deltaMACG_f) -> Sum/1
  r8x3RA_f/1 -> MATLAB Function/1(r8x3RA_f)
  r8x3MAARP_f/1 -> Sum/2

== matlab function FMmodelBasic/LSA_02_Fmmodel/aircraft/5_aerodynamics/52_wing_and_fuselage/524_aerodynamic_moments/5242_with_respect_to_CG/MATLAB Function ==
  data: r8x3RA_f input; aeroDB parameter; r8x3deltaMACG_f output size=[3,1]
function r8x3deltaMACG_f = momentCalcCG(r8x3RA_f,aeroDB)

r8x3rARP_f = [aeroDB.xARP_f;aeroDB.yARP_f;aeroDB.zARP_f];
r8x3deltaMACG_f = cross(r8x3rARP_f,r8x3RA_f); % moment yang bekerja hanya akan menambahkan komponen pitching moment. hal ini disebabkan karena perbedaan lokasi CG dan Aerodynamic center hanya mempengaruhi pitching moment

== matlab function FMmodelBasic/LSA_02_Fmmodel/aircraft/8_equations_of_motion/83_attitude_equation/MATLAB Function ==
  data: r8x3attitude input; r8x3attitudeDot output size=[3,1]; r8x3om_f input
function r8x3attitudeDot = fcn(r8x3attitude,r8x3om_f)

r8phi = r8x3attitude(1);
r8th = r8x3attitude(2);


r8T_phf = [1 sin(r8phi)*tan(r8th) cos(r8phi)*tan(r8th);0 cos(r8phi) -sin(r8phi);0 sin(r8phi)/cos(r8th) cos(r8phi)/cos(r8th)];

r8x3attitudeDot = r8T_phf * r8x3om_f;

== matlab function FMmodelBasic/LSA_02_Fmmodel/aircraft/8_equations_of_motion/82_translational_equation/MATLAB Function ==
  data: r8x3om_f input; r8x3VK_f input; r8mOEW input; r8x3VK_fDot output size=[3,1]; r8x3R_f input
function r8x3VK_fDot  = fcn(r8x3om_f,r8x3VK_f,r8mOEW,r8x3R_f)
%#codegen


r8x3VK_fDot = (r8x3R_f/r8mOEW)+(cross(-r8x3om_f,r8x3VK_f));

== matlab function FMmodelBasic/LSA_02_Fmmodel/aircraft/1_inertial_properties/MATLAB Function ==
  data: r8Ixx_f input; r8x3x3I_f output; r8Iyy_f input; r8Izz_f input; r8Ixy_f input; r8Ixz_f input; r8Iyz_f input
function r8x3x3I_f = fcn(r8Ixx_f,r8Iyy_f,r8Izz_f,r8Ixy_f,r8Ixz_f,r8Iyz_f)
%#codegen

r8x3x3I_f = [r8Ixx_f -r8Ixy_f -r8Ixz_f;-r8Ixy_f r8Iyy_f -r8Iyz_f;-r8Ixz_f -r8Iyz_f r8Izz_f];

== matlab function FMmodelBasic/LSA_02_Fmmodel/aircraft/5_aerodynamics/51_effective_flow_at_ARP/513_aerodynamic_to_bodyfixed/Tfa ==
  data: r8alARP input; r8T_fa output; r8beARP input
function r8T_fa = trans_fa(r8alARP,r8beARP)
%#codegen

r8T_fa = [cos(r8alARP)*cos(r8beARP) -cos(r8alARP)*sin(r8beARP) -sin(r8alARP);sin(r8beARP) cos(r8beARP) 0;sin(r8alARP)*cos(r8beARP) -sin(r8alARP)*sin(r8beARP) cos(r8alARP)];

== matlab function FMmodelBasic/LSA_02_Fmmodel/aircraft/5_aerodynamics/52_wing_and_fuselage/524_aerodynamic_moments/5241_with_respect_to_ARP/MATLAB Function ==
  data: r8Pdyn input; r8x3mcoef input; aeroDB parameter; r8x3MAARP_f output size=[3,1]
function r8x3MAARP_f = momentCalcARP(r8Pdyn,r8x3mcoef,aeroDB)

r8x3MAARP_f = zeros(3,1);
r8x3MAARP_f(1) = r8x3mcoef(1)*r8Pdyn*aeroDB.S*aeroDB.b*0.5;
r8x3MAARP_f(2) = r8x3mcoef(2)*r8Pdyn*aeroDB.S*aeroDB.lmu;
r8x3MAARP_f(3) = r8x3mcoef(3)*r8Pdyn*aeroDB.S*aeroDB.b*0.5;

== matlab function FMmodelBasic/LSA_02_Fmmodel/aircraft/5_aerodynamics/52_wing_and_fuselage/ 523_aerodynamic_forces/5231_in_aerodynamic_coordinates/MATLAB Function ==
  data: r8Pdyn input; r8x3RA_a output size=[3,1]; r8x3forceCoef input; aeroDB parameter
function r8x3RA_a = forceCalc(r8Pdyn,r8x3forceCoef,aeroDB)

W = r8Pdyn*aeroDB.S*-r8x3forceCoef(1);
Q = r8Pdyn*aeroDB.S*r8x3forceCoef(2);
A = r8Pdyn*aeroDB.S*-r8x3forceCoef(3);

r8x3RA_a = [W;Q;A];

== matlab function FMmodelBasic/LSA_02_Fmmodel/aircraft/5_aerodynamics/52_wing_and_fuselage/522_aerodynamic_coefficients/MATLAB Function ==
  data: r8x3forceCoef output size=[3,1]; r8x3momentCoef output size=[3,1]; AeroVar input; aeroDB parameter
function [r8x3forceCoef,r8x3momentCoef] = AeroForceMoment(AeroVar,aeroDB)

% ======================= SHORT OPTIMIZED FUNCTION ====================== %
AeroVarExtLon = [AeroVar;AeroVar.^2;AeroVar.^3];
AeroVarExtLat = AeroVarExtLon;
% Accounting for symmetry (aeroDB.sym=[2 3 5 7 8])
AeroVarExtLon(1,aeroDB.sim)=AeroVarExtLon(1,aeroDB.sim).*sign(AeroVar(aeroDB.sim));
AeroVarExtLon(3,aeroDB.sim)=AeroVarExtLon(3,aeroDB.sim).*sign(AeroVar(aeroDB.sim));
AeroVarExtLat(2,aeroDB.sim)=AeroVarExtLat(2,aeroDB.sim).*sign(AeroVar(aeroDB.sim));
% Reshaping the AeroVarExt to the matrix value [1;AeroVarExt]
AeroVarExtLon = [1;AeroVarExtLon(:)];
AeroVarExtLat = [1;AeroVarExtLat(:)];
% Calculation for the aerodynamic coefficient
CA = AeroVarExtLon'*aeroDB.coefCA*AeroVarExtLon;
CW = AeroVarExtLon'*aeroDB.coefCW*AeroVarExtLon;
Cm = AeroVarExtLon'*aeroDB.coefCm*AeroVarExtLon;
Cl = AeroVarExtLat'*aeroDB.coefCl*AeroVarExtLat;
Cn = AeroVarExtLat'*aeroDB.coefCn*AeroVarExtLat;
CQ = AeroVarExtLat'*aeroDB.coefCQ*AeroVarExtLat;
r8x3forceCoef = [CW;CQ;CA];
r8x3momentCoef = [Cl;Cm;Cn];
end
% ======================================================================= %
% ============================ OLD FUNCTION ============================= %
% % a Matlab function which returns the 6 aerodynamic coefficients a output variables, 
% % using as an Input the vector of dimensionless influence variables (Pi-factors) as well 
% % as the aerodynamic database. Use the presented matrix multiplication scheme for the calculation. 
% % See equation 12 to 15 to create this function
% 
% AeroVarExtCA = [AeroVar;AeroVar.^2;AeroVar.^3];
% AeroVarExtCW = AeroVarExtCA;
% AeroVarExtCQ = AeroVarExtCA;
% AeroVarExtCL = AeroVarExtCA;
% AeroVarExtCM = AeroVarExtCA;
% AeroVarExtCN = AeroVarExtCA;
% 
% % aeroDB.asimCA = [fals,true,true,false,true,false,true,true,false,false];
% % AeroVarExt(1,[2,3,5,7,8])*sign(AeroVar([2,3,5,7,8])) % number
% % indexing,choice the true ones, in aeroDB.asimCA
% 
% % FOR LONGITUDINAL COEFFICIENT
% AeroVarExtCA (1,aeroDB.asimCA) = AeroVarExtCA(1,aeroDB.asimCA).*sign(AeroVar(aeroDB.asimCA)); % logical indexing, in the left hand side is 1 row 5 coulumn
% AeroVarExtCA (3,aeroDB.asimCA) = AeroVarExtCA(3,aeroDB.asimCA).*sign(AeroVar(aeroDB.asimCA));
% AeroVarExtCA (2,aeroDB.osimCA) = AeroVarExtCA(2,aeroDB.osimCA).*sign(AeroVar(aeroDB.osimCA));
% AeroVarExtCW (1,aeroDB.asimCW) = AeroVarExtCW(1,aeroDB.asimCW).*sign(AeroVar(aeroDB.asimCW)); 
% AeroVarExtCW (3,aeroDB.asimCW) = AeroVarExtCW(3,aeroDB.asimCW).*sign(AeroVar(aeroDB.asimCW));
% AeroVarExtCW (2,aeroDB.osimCW) = AeroVarExtCW(2,aeroDB.osimCW).*sign(AeroVar(aeroDB.osimCW));
% AeroVarExtCM (1,aeroDB.asimCM) = AeroVarExtCM(1,aeroDB.asimCM).*sign(AeroVar(aeroDB.asimCM)); 
% AeroVarExtCM (3,aeroDB.asimCM) = AeroVarExtCM(3,aeroDB.asimCM).*sign(AeroVar(aeroDB.asimCM));
% AeroVarExtCM (2,aeroDB.osimCM) = AeroVarExtCM(2,aeroDB.osimCM).*sign(AeroVar(aeroDB.osimCM));
% 
% % FOR LATERAL COEFFICIENT
% AeroVarExtCL (1,aeroDB.asimCL) = AeroVarExtCL(1,aeroDB.asimCL).*sign(AeroVar(aeroDB.asimCL)); % logical indexing, in the left hand side is 1 row 5 coulumn
% AeroVarExtCL (3,aeroDB.asimCL) = AeroVarExtCL(3,aeroDB.asimCL).*sign(AeroVar(aeroDB.asimCL));
% AeroVarExtCL (2,aeroDB.osimCL) = AeroVarExtCL(2,aeroDB.osimCL).*sign(AeroVar(aeroDB.osimCL));
% AeroVarExtCN (1,aeroDB.asimCN) = AeroVarExtCN(1,aeroDB.asimCN).*sign(AeroVar(aeroDB.asimCN)); 
% AeroVarExtCN (3,aeroDB.asimCN) = AeroVarExtCN(3,aeroDB.asimCN).*sign(AeroVar(aeroDB.asimCN));
% AeroVarExtCN (2,aeroDB.osimCN) = AeroVarExtCN(2,aeroDB.osimCN).*sign(AeroVar(aeroDB.osimCN));
% AeroVarExtCQ (1,aeroDB.asimCQ) = AeroVarExtCQ(1,aeroDB.asimCQ).*sign(AeroVar(aeroDB.asimCQ)); 
% AeroVarExtCQ (3,aeroDB.asimCQ) = AeroVarExtCQ(3,aeroDB.asimCQ).*sign(AeroVar(aeroDB.asimCQ));
% AeroVarExtCQ (2,aeroDB.osimCQ) = AeroVarExtCQ(2,aeroDB.osimCQ).*sign(AeroVar(aeroDB.osimCQ));
% 
% % Reshaping the AeroVarExt to the matrix value [1;AeroVarExt]
% AeroVarExtCA = [1;AeroVarExtCA(:)];
% AeroVarExtCW = [1;AeroVarExtCW(:)];
% AeroVarExtCM = [1;AeroVarExtCM(:)];
% AeroVarExtCL = [1;AeroVarExtCL(:)];
% AeroVarExtCN = [1;AeroVarExtCN(:)];
% AeroVarExtCQ = [1;AeroVarExtCQ(:)];
% 
% % Calculation for the aerodynamic coefficient
% CA = AeroVarExtCA'*aeroDB.coefCA*AeroVarExtCA;
% CW = AeroVarExtCW'*aeroDB.coefCW*AeroVarExtCW;
% CM = AeroVarExtCM'*aeroDB.coefCM*AeroVarExtCM;
% CL = AeroVarExtCL'*aeroDB.coefCL*AeroVarExtCL;
% CN = AeroVarExtCN'*aeroDB.coefCN*AeroVarExtCN;
% CQ = AeroVarExtCQ'*aeroDB.coefCQ*AeroVarExtCQ;
% 
% 
% % AeroVarExt(1,2)*sign(AeroVar(2))
% % AeroVarExt(1,3)*sign(AeroVar(3))
% % AeroVarExt(1,5)*sign(AeroVar(5))
% % AeroVarExt(1,7)*sign(AeroVar(7))
% % AeroVarExt(1,8)*sign(AeroVar(8))
% end

== matlab function FMmodelBasic/LSA_02_Fmmodel/aircraft/4_environment/41_atmosphere/411_ISA_conditions/4113_static_pressure/MATLAB Function For Calculated P ==
  data: T input; H input; r8Pstat output; T0 input; H0 input; P0 input; envDB parameter
function r8Pstat  = fcn(T,H,T0,H0,P0,envDB)

if abs(T-T0)>eps     %constant gradient
    k=(T-T0)/(H-H0);
    r8Pstat=P0*((T/T0)^(-envDB.g/(k*envDB.R)));
else                        %constant temperature
    r8Pstat=P0*exp(-envDB.g/(envDB.R*T0)*(H-H0));
end
end

== matlab function FMmodelBasic/LSA_02_Fmmodel/aircraft/8_equations_of_motion/84_rotational_equation/MATLAB Function ==
  data: r8x3om_f input; r8x3om_fDot output size=[3,1]; r8x3x3I_f input; r8x3M_f input
function r8x3om_fDot = crossAngCalc(r8x3om_f,r8x3x3I_f, r8x3M_f)
%#codegen

r8x3om_fDot = r8x3x3I_f\(r8x3M_f + cross(-r8x3om_f,r8x3x3I_f*r8x3om_f));
